simulink model "ball_beam_simulink"  (R2020a)
settings: Solver=VariableStepAuto  StartTime=0.0  StopTime=10  FixedStep=0.01  MaxStep=0.01  RelTol=1e-10
values from neighbouring files (symbols this model uses):
  k = (DATI.m*DATI.g*DATI.d) / (m_eq * DATI.L)    [prova_regolatore.m]
settings Model: NumberOfSteps=3  Creator=peter  LastModifiedBy=peter
settings SolverCC: ShapePreserveControl=EnableAll  ZeroCrossAlgorithm=Adaptive
settings DataIOCC: ExternalInput=[t]  SaveFormat=Array  SignalLogging=off  DSMLogging=off  ReturnWorkspaceOutputs=off  DatasetSignalFormat=timetable

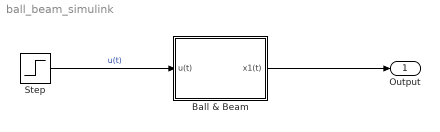
== system ball_beam_simulink ==
  Ball & Beam : Subsystem  VariantControl=Choice
  Step : Step  Time=0  SampleTime=0
  Output : Outport  SignalName=y(t)
  wires:
  Step/1 -> Ball & Beam/1(u(t))  "u(t)"
  Ball & Beam/1(x1(t)) -> Output/1

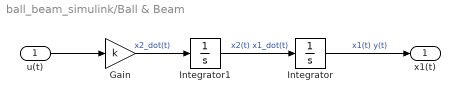
== system ball_beam_simulink/Ball & Beam ==
  u(t) : Inport
  Gain : Gain  Gain=k
  Integrator : Integrator
  Integrator1 : Integrator
  x1(t) : Outport
  wires:
  Integrator/1 -> x1(t)/1  "x1(t) y(t)"
  u(t)/1 -> Gain/1
  Integrator1/1 -> Integrator/1  "x2(t) x1_dot(t)"
  Gain/1 -> Integrator1/1  "x2_dot(t)"
